simulink library "see_saw_princess"  (R2013b)
settings: Solver=ode45  StartTime=0.0  StopTime=10.0  RelTol=1e-3
undefined symbols (not defined in the file): DiscIntNeverNeededParam, K, R
libraries: legonxtlib x4
settings Model: Creator=mbiesiad  LastModifiedBy=pvinnako

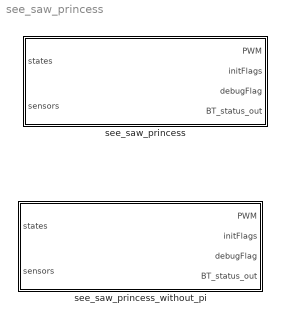
== system see_saw_princess ==
  see_saw_princess : Stateflow chart  TreatAsAtomicUnit=on
  see_saw_princess_without_pi : Stateflow chart  TreatAsAtomicUnit=on

== system see_saw_princess/see_saw_princess/see_saw_mode.DispVar ==
  Var : Inport  OutDataTypeStr=single  PortDimensions=1
  f : TriggerPort  TriggerType=function-call
      settings: CopyFcn=Stateflow.SLINSF.SimulinkMan.removeBlockPreDeleteFcn  PreDeleteFcn=Stateflow.SLINSF.SimulinkMan.unsafePredeleteFcn
  Gain : Gain  Gain=100
  LCD : legonxtlib/LCD  slcdStr=Light  slcdLine=2  slcdFormat=Decimal
  wires:
  Gain/1 -> LCD/1
  Var/1 -> Gain/1

== system see_saw_princess/see_saw_princess/see_saw_mode.Speak ==
  f : TriggerPort  TriggerType=function-call
      settings: CopyFcn=Stateflow.SLINSF.SimulinkMan.removeBlockPreDeleteFcn  PreDeleteFcn=Stateflow.SLINSF.SimulinkMan.unsafePredeleteFcn
  Constant : Constant  Value=50
  Speaker : legonxtlib/Speaker  sinputMode=Volume only  sspeakerFreq=800  sspeakerVolume=50  sspeakerDuration=100
  wires:
  Constant/1 -> Speaker/1

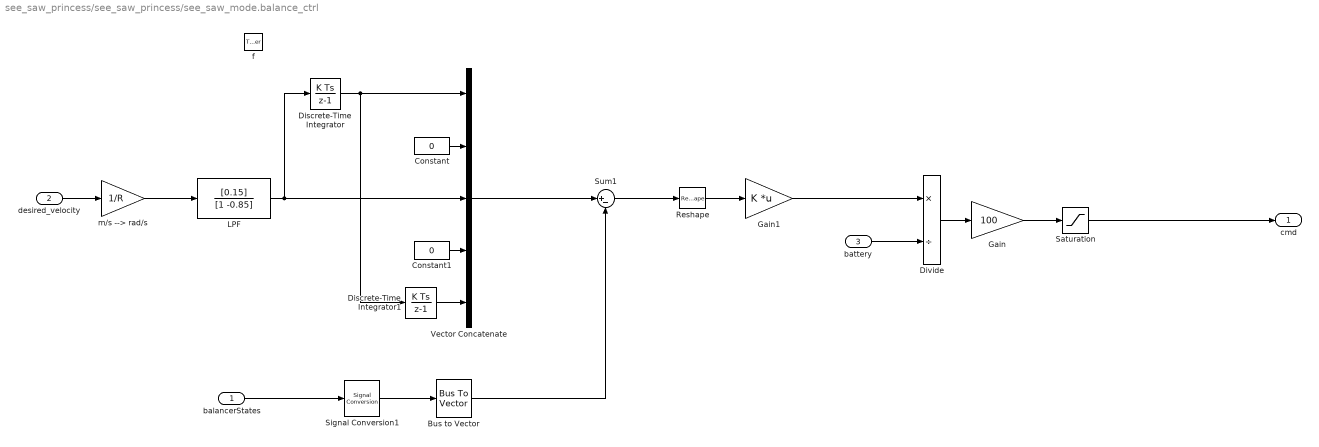
== system see_saw_princess/see_saw_princess/see_saw_mode.balance_ctrl ==
  balancerStates : Inport  OutDataTypeStr=Bus: Balancer_States_Bus  PortDimensions=1
  desired_velocity : Inport  Port=2  OutDataTypeStr=single  PortDimensions=1  BusOutputAsStruct=on
  battery : Inport  Port=3  OutDataTypeStr=double  PortDimensions=1
  f : TriggerPort  TriggerType=function-call
      settings: CopyFcn=Stateflow.SLINSF.SimulinkMan.removeBlockPreDeleteFcn  PreDeleteFcn=Stateflow.SLINSF.SimulinkMan.unsafePredeleteFcn
  Bus to Vector : BusToVector
  Constant : Constant  Value=0  OutDataTypeStr=single
  Constant1 : Constant  Value=0  OutDataTypeStr=single
  Discrete-Time Integrator : DiscreteIntegrator  SampleTime=-1  ICPrevOutput=DiscIntNeverNeededParam  ICPrevScaledInput=DiscIntNeverNeededParam
  Discrete-Time Integrator1 : DiscreteIntegrator  SampleTime=-1  ICPrevOutput=DiscIntNeverNeededParam  ICPrevScaledInput=DiscIntNeverNeededParam
  Divide : Product  Inputs=*/
  Gain : Gain  Gain=100
  Gain1 : Gain  Gain=K  Multiplication=Matrix(K*u)
  LPF : DiscreteFilter  Numerator=[0.15]  Denominator=[1 -0.85]
  Reshape : Reshape  OutputDimensionality=Column vector (2-D)
  Saturation : Saturate  UpperLimit=100  LowerLimit=-100  OutDataTypeStr=single
  Signal Conversion1 : SignalConversion  ConversionOutput=Virtual bus
  Sum1 : Sum  Inputs=|+-
  Vector Concatenate : Concatenate  NumInputs=5
  m/s --> rad/s : Gain  Gain=1/R
  cmd : Outport  OutDataTypeStr=single  PortDimensions=1  InitialOutput=0
  wires:
  Discrete-Time Integrator1/1 -> Vector Concatenate/5
  Discrete-Time Integrator/1 -> Vector Concatenate/1, Discrete-Time Integrator1/1
  Constant1/1 -> Vector Concatenate/4
  LPF/1 -> Vector Concatenate/3, Discrete-Time Integrator/1
  Constant/1 -> Vector Concatenate/2
  m/s --> rad/s/1 -> LPF/1
  Signal Conversion1/1 -> Bus to Vector/1
  Divide/1 -> Gain/1
  Gain/1 -> Saturation/1
  Gain1/1 -> Divide/1
  Saturation/1 -> cmd/1
  battery/1 -> Divide/2
  Vector Concatenate/1 -> Sum1/1
  balancerStates/1 -> Signal Conversion1/1
  Bus to Vector/1 -> Sum1/2
  desired_velocity/1 -> m/s --> rad/s/1
  Sum1/1 -> Reshape/1
  Reshape/1 -> Gain1/1

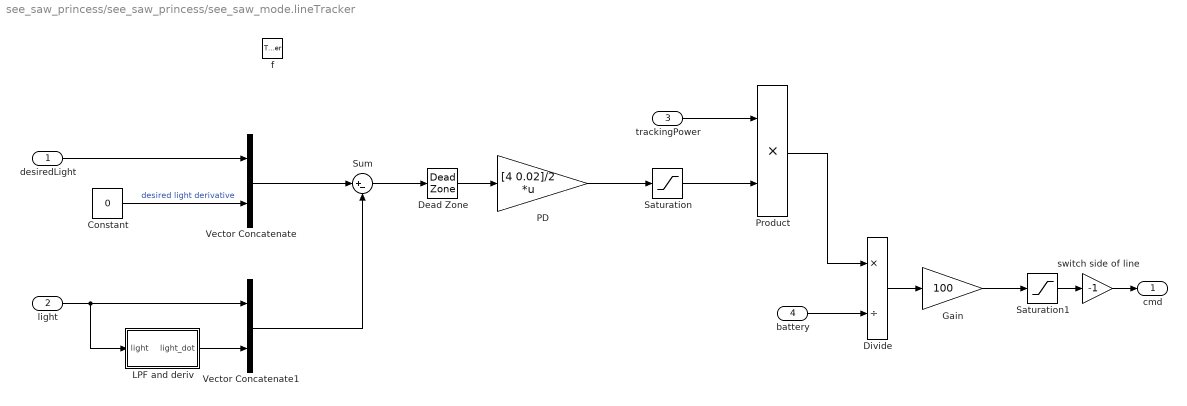
== system see_saw_princess/see_saw_princess/see_saw_mode.lineTracker ==
  desiredLight : Inport  OutDataTypeStr=single  PortDimensions=1
  light : Inport  Port=2  OutDataTypeStr=single  PortDimensions=1
  trackingPower : Inport  Port=3  OutDataTypeStr=single  PortDimensions=1
  battery : Inport  Port=4  OutDataTypeStr=double  PortDimensions=1
  f : TriggerPort  TriggerType=function-call
      settings: CopyFcn=Stateflow.SLINSF.SimulinkMan.removeBlockPreDeleteFcn  PreDeleteFcn=Stateflow.SLINSF.SimulinkMan.unsafePredeleteFcn
  Constant : Constant  Value=0  OutDataTypeStr=single
  Dead Zone : DeadZone  LowerValue=-0.02  UpperValue=0.02  SaturateOnIntegerOverflow=on
  Divide : Product  Inputs=*/
  Gain : Gain  Gain=100
  LPF and deriv : Subsystem
  PD : Gain  Gain="[4  0.02]/2"  Multiplication=Matrix(K*u)
  Product : Product
  Saturation : Saturate  UpperLimit=6  LowerLimit=-6
  Saturation1 : Saturate  UpperLimit=100  LowerLimit=-100  OutDataTypeStr=single
  Sum : Sum  Inputs=|+-
  Vector Concatenate : Concatenate
  Vector Concatenate1 : Concatenate
  switch side of line : Gain  Gain=-1
  cmd : Outport  OutDataTypeStr=single  PortDimensions=1
  wires:
  Saturation1/1 -> switch side of line/1
  Divide/1 -> Gain/1
  Gain/1 -> Saturation1/1
  battery/1 -> Divide/2
  Product/1 -> Divide/1
  trackingPower/1 -> Product/1
  Saturation/1 -> Product/2
  PD/1 -> Saturation/1
  Dead Zone/1 -> PD/1
  Sum/1 -> Dead Zone/1
  Vector Concatenate1/1 -> Sum/2
  Vector Concatenate/1 -> Sum/1
  light/1 -> Vector Concatenate1/1, LPF and deriv/1(light)
  LPF and deriv/1(light_dot) -> Vector Concatenate1/2
  Constant/1 -> Vector Concatenate/2  "desired light derivative"
  desiredLight/1 -> Vector Concatenate/1
  switch side of line/1 -> cmd/1

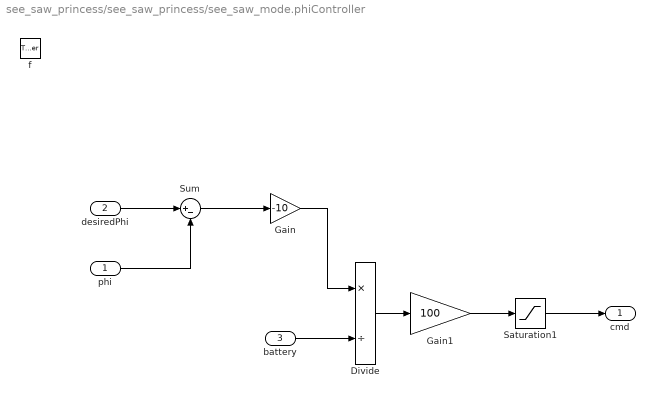
== system see_saw_princess/see_saw_princess/see_saw_mode.phiController ==
  phi : Inport  OutDataTypeStr=single  PortDimensions=1
  desiredPhi : Inport  Port=2  OutDataTypeStr=single  PortDimensions=1
  battery : Inport  Port=3  OutDataTypeStr=double  PortDimensions=1
  f : TriggerPort  TriggerType=function-call
      settings: CopyFcn=Stateflow.SLINSF.SimulinkMan.removeBlockPreDeleteFcn  PreDeleteFcn=Stateflow.SLINSF.SimulinkMan.unsafePredeleteFcn
  Divide : Product  Inputs=*/
  Gain : Gain  Gain=-10
  Gain1 : Gain  Gain=100
  Saturation1 : Saturate  UpperLimit=100  LowerLimit=-100  OutDataTypeStr=single
  Sum : Sum  Inputs=|+-
  cmd : Outport
  wires:
  Saturation1/1 -> cmd/1
  Gain/1 -> Divide/1
  Divide/1 -> Gain1/1
  Gain1/1 -> Saturation1/1
  battery/1 -> Divide/2
  Sum/1 -> Gain/1
  phi/1 -> Sum/2
  desiredPhi/1 -> Sum/1

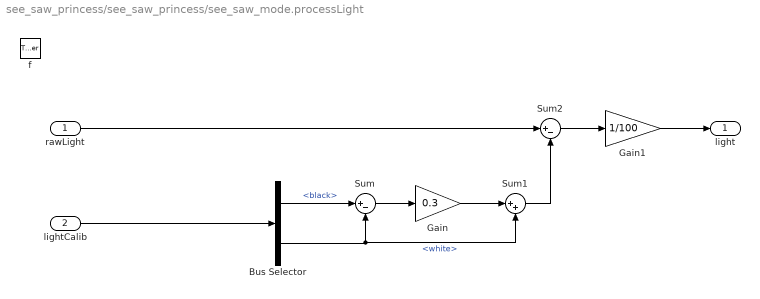
== system see_saw_princess/see_saw_princess/see_saw_mode.processLight ==
  rawLight : Inport  OutDataTypeStr=single  PortDimensions=1
  lightCalib : Inport  Port=2  OutDataTypeStr=Bus: Light_Bus  PortDimensions=1
  f : TriggerPort  TriggerType=function-call
      settings: CopyFcn=Stateflow.SLINSF.SimulinkMan.removeBlockPreDeleteFcn  PreDeleteFcn=Stateflow.SLINSF.SimulinkMan.unsafePredeleteFcn
  Bus Selector : BusSelector  OutputSignals=black,white
  Gain : Gain  Gain=0.3
  Gain1 : Gain  Gain=1/100
  Sum : Sum  Inputs=|+-
  Sum1 : Sum  Inputs=|++
  Sum2 : Sum  Inputs=|+-
  light : Outport
  wires:
  Gain1/1 -> light/1
  Sum2/1 -> Gain1/1
  Sum1/1 -> Sum2/2
  rawLight/1 -> Sum2/1
  Gain/1 -> Sum1/1
  Sum/1 -> Gain/1
  Bus Selector/2 -> Sum/2, Sum1/2  "<white>"
  Bus Selector/1 -> Sum/1  "<black>"
  lightCalib/1 -> Bus Selector/1

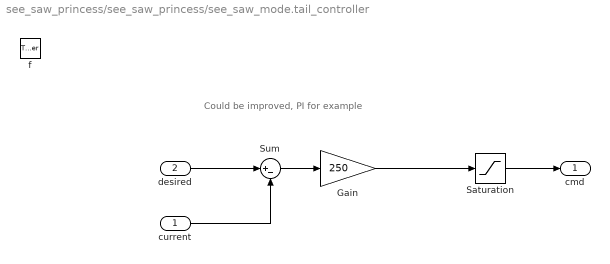
== system see_saw_princess/see_saw_princess/see_saw_mode.tail_controller ==
  note: Could be improved, PI for example
  current : Inport  OutDataTypeStr=single  PortDimensions=1
  desired : Inport  Port=2  OutDataTypeStr=single  PortDimensions=1
  f : TriggerPort  TriggerType=function-call
      settings: CopyFcn=Stateflow.SLINSF.SimulinkMan.removeBlockPreDeleteFcn  PreDeleteFcn=Stateflow.SLINSF.SimulinkMan.unsafePredeleteFcn
  Gain : Gain  Gain=250
  Saturation : Saturate  UpperLimit=100  LowerLimit=-100  OutDataTypeStr=single
  Sum : Sum  Inputs=|+-
  cmd : Outport  OutDataTypeStr=single  PortDimensions=1  InitialOutput=0
  wires:
  Saturation/1 -> cmd/1
  Gain/1 -> Saturation/1
  desired/1 -> Sum/1
  current/1 -> Sum/2
  Sum/1 -> Gain/1

== system see_saw_princess/see_saw_princess_without_pi/see_saw_mode.DispVar ==
  Var : Inport  OutDataTypeStr=single  PortDimensions=1
  f : TriggerPort  TriggerType=function-call
      settings: CopyFcn=Stateflow.SLINSF.SimulinkMan.removeBlockPreDeleteFcn  PreDeleteFcn=Stateflow.SLINSF.SimulinkMan.unsafePredeleteFcn
  Gain : Gain  Gain=100
  LCD : legonxtlib/LCD  slcdStr=Light  slcdLine=2  slcdFormat=Decimal
  wires:
  Var/1 -> Gain/1
  Gain/1 -> LCD/1

== system see_saw_princess/see_saw_princess_without_pi/see_saw_mode.Speak ==
  f : TriggerPort  TriggerType=function-call
      settings: CopyFcn=Stateflow.SLINSF.SimulinkMan.removeBlockPreDeleteFcn  PreDeleteFcn=Stateflow.SLINSF.SimulinkMan.unsafePredeleteFcn
  Constant : Constant  Value=50
  Speaker : legonxtlib/Speaker  sinputMode=Volume only  sspeakerFreq=800  sspeakerVolume=50  sspeakerDuration=100
  wires:
  Constant/1 -> Speaker/1

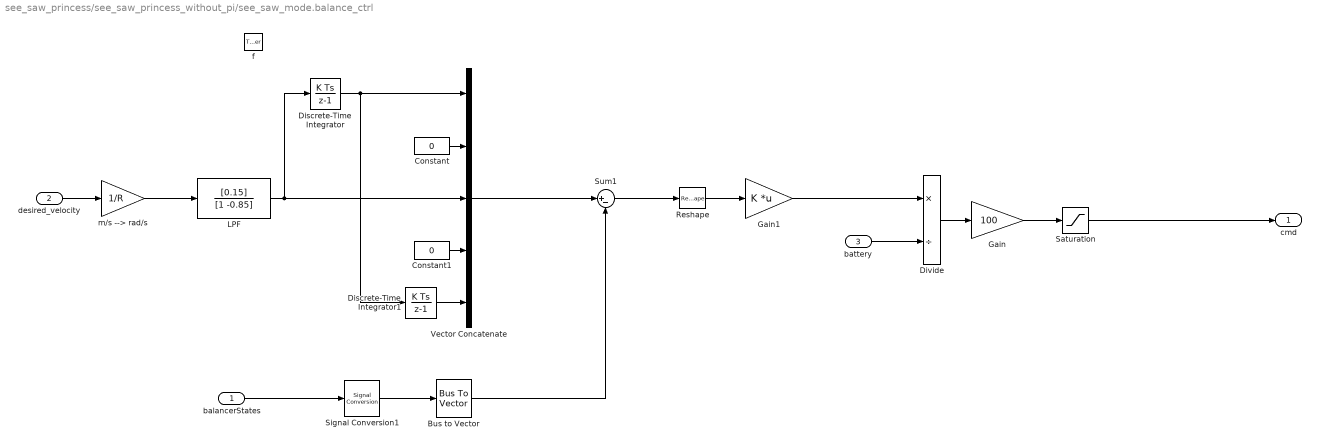
== system see_saw_princess/see_saw_princess_without_pi/see_saw_mode.balance_ctrl ==
  balancerStates : Inport  OutDataTypeStr=Bus: Balancer_States_Bus  PortDimensions=1
  desired_velocity : Inport  Port=2  OutDataTypeStr=single  PortDimensions=1  BusOutputAsStruct=on
  battery : Inport  Port=3  OutDataTypeStr=double  PortDimensions=1
  f : TriggerPort  TriggerType=function-call
      settings: CopyFcn=Stateflow.SLINSF.SimulinkMan.removeBlockPreDeleteFcn  PreDeleteFcn=Stateflow.SLINSF.SimulinkMan.unsafePredeleteFcn
  Bus to Vector : BusToVector
  Constant : Constant  Value=0  OutDataTypeStr=single
  Constant1 : Constant  Value=0  OutDataTypeStr=single
  Discrete-Time Integrator : DiscreteIntegrator  SampleTime=-1  ICPrevOutput=DiscIntNeverNeededParam  ICPrevScaledInput=DiscIntNeverNeededParam
  Discrete-Time Integrator1 : DiscreteIntegrator  SampleTime=-1  ICPrevOutput=DiscIntNeverNeededParam  ICPrevScaledInput=DiscIntNeverNeededParam
  Divide : Product  Inputs=*/
  Gain : Gain  Gain=100
  Gain1 : Gain  Gain=K  Multiplication=Matrix(K*u)
  LPF : DiscreteFilter  Numerator=[0.15]  Denominator=[1 -0.85]
  Reshape : Reshape  OutputDimensionality=Column vector (2-D)
  Saturation : Saturate  UpperLimit=100  LowerLimit=-100  OutDataTypeStr=single
  Signal Conversion1 : SignalConversion  ConversionOutput=Virtual bus
  Sum1 : Sum  Inputs=|+-
  Vector Concatenate : Concatenate  NumInputs=5
  m/s --> rad/s : Gain  Gain=1/R
  cmd : Outport  OutDataTypeStr=single  PortDimensions=1  InitialOutput=0
  wires:
  Reshape/1 -> Gain1/1
  Sum1/1 -> Reshape/1
  desired_velocity/1 -> m/s --> rad/s/1
  Bus to Vector/1 -> Sum1/2
  balancerStates/1 -> Signal Conversion1/1
  Vector Concatenate/1 -> Sum1/1
  battery/1 -> Divide/2
  Saturation/1 -> cmd/1
  Gain1/1 -> Divide/1
  Gain/1 -> Saturation/1
  Divide/1 -> Gain/1
  Signal Conversion1/1 -> Bus to Vector/1
  m/s --> rad/s/1 -> LPF/1
  Constant/1 -> Vector Concatenate/2
  LPF/1 -> Discrete-Time Integrator/1, Vector Concatenate/3
  Constant1/1 -> Vector Concatenate/4
  Discrete-Time Integrator/1 -> Discrete-Time Integrator1/1, Vector Concatenate/1
  Discrete-Time Integrator1/1 -> Vector Concatenate/5

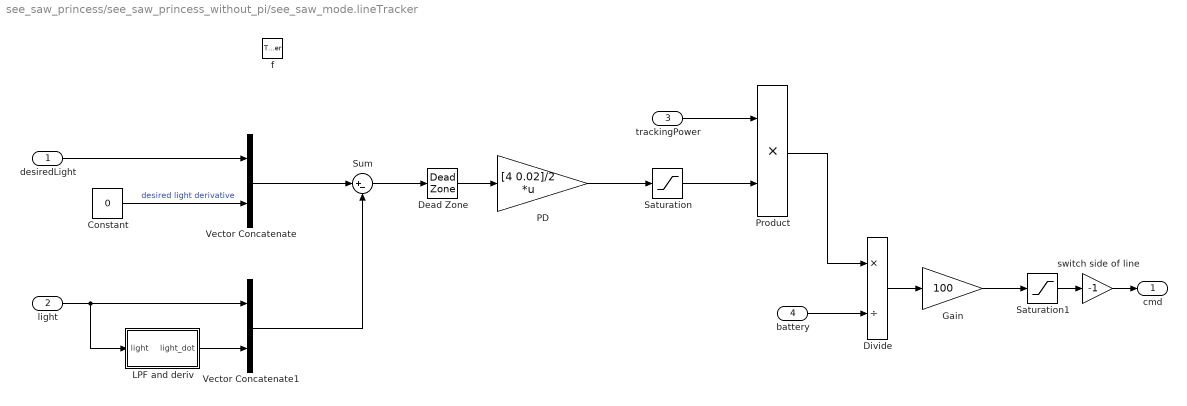
== system see_saw_princess/see_saw_princess_without_pi/see_saw_mode.lineTracker ==
  desiredLight : Inport  OutDataTypeStr=single  PortDimensions=1
  light : Inport  Port=2  OutDataTypeStr=single  PortDimensions=1
  trackingPower : Inport  Port=3  OutDataTypeStr=single  PortDimensions=1
  battery : Inport  Port=4  OutDataTypeStr=double  PortDimensions=1
  f : TriggerPort  TriggerType=function-call
      settings: CopyFcn=Stateflow.SLINSF.SimulinkMan.removeBlockPreDeleteFcn  PreDeleteFcn=Stateflow.SLINSF.SimulinkMan.unsafePredeleteFcn
  Constant : Constant  Value=0  OutDataTypeStr=single
  Dead Zone : DeadZone  LowerValue=-0.02  UpperValue=0.02  SaturateOnIntegerOverflow=on
  Divide : Product  Inputs=*/
  Gain : Gain  Gain=100
  LPF and deriv : Subsystem
  PD : Gain  Gain="[4  0.02]/2"  Multiplication=Matrix(K*u)
  Product : Product
  Saturation : Saturate  UpperLimit=6  LowerLimit=-6
  Saturation1 : Saturate  UpperLimit=100  LowerLimit=-100  OutDataTypeStr=single
  Sum : Sum  Inputs=|+-
  Vector Concatenate : Concatenate
  Vector Concatenate1 : Concatenate
  switch side of line : Gain  Gain=-1
  cmd : Outport  OutDataTypeStr=single  PortDimensions=1
  wires:
  switch side of line/1 -> cmd/1
  desiredLight/1 -> Vector Concatenate/1
  Constant/1 -> Vector Concatenate/2  "desired light derivative"
  LPF and deriv/1(light_dot) -> Vector Concatenate1/2
  light/1 -> LPF and deriv/1(light), Vector Concatenate1/1
  Vector Concatenate/1 -> Sum/1
  Vector Concatenate1/1 -> Sum/2
  Sum/1 -> Dead Zone/1
  Dead Zone/1 -> PD/1
  PD/1 -> Saturation/1
  Saturation/1 -> Product/2
  trackingPower/1 -> Product/1
  Product/1 -> Divide/1
  battery/1 -> Divide/2
  Gain/1 -> Saturation1/1
  Divide/1 -> Gain/1
  Saturation1/1 -> switch side of line/1

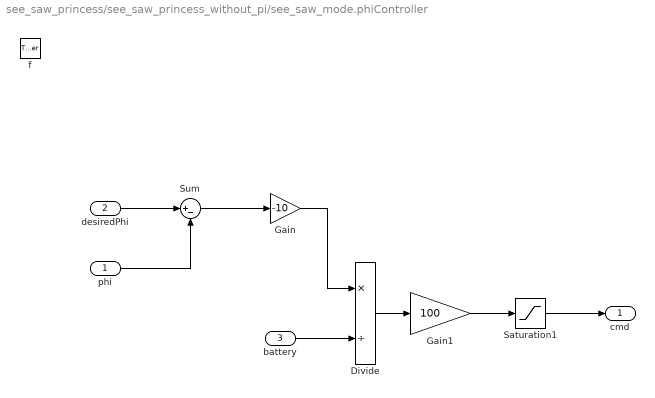
== system see_saw_princess/see_saw_princess_without_pi/see_saw_mode.phiController ==
  phi : Inport  OutDataTypeStr=single  PortDimensions=1
  desiredPhi : Inport  Port=2  OutDataTypeStr=single  PortDimensions=1
  battery : Inport  Port=3  OutDataTypeStr=double  PortDimensions=1
  f : TriggerPort  TriggerType=function-call
      settings: CopyFcn=Stateflow.SLINSF.SimulinkMan.removeBlockPreDeleteFcn  PreDeleteFcn=Stateflow.SLINSF.SimulinkMan.unsafePredeleteFcn
  Divide : Product  Inputs=*/
  Gain : Gain  Gain=-10
  Gain1 : Gain  Gain=100
  Saturation1 : Saturate  UpperLimit=100  LowerLimit=-100  OutDataTypeStr=single
  Sum : Sum  Inputs=|+-
  cmd : Outport
  wires:
  desiredPhi/1 -> Sum/1
  phi/1 -> Sum/2
  Sum/1 -> Gain/1
  battery/1 -> Divide/2
  Gain1/1 -> Saturation1/1
  Divide/1 -> Gain1/1
  Gain/1 -> Divide/1
  Saturation1/1 -> cmd/1

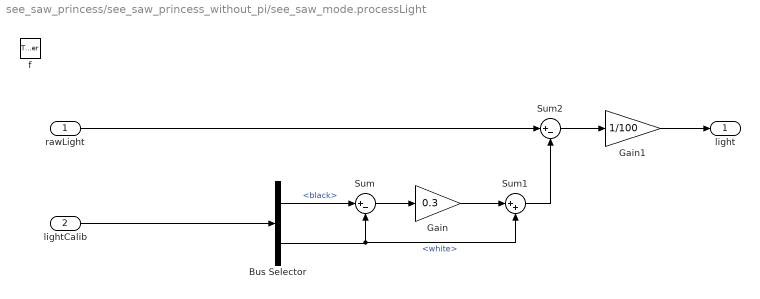
== system see_saw_princess/see_saw_princess_without_pi/see_saw_mode.processLight ==
  rawLight : Inport  OutDataTypeStr=single  PortDimensions=1
  lightCalib : Inport  Port=2  OutDataTypeStr=Bus: Light_Bus  PortDimensions=1
  f : TriggerPort  TriggerType=function-call
      settings: CopyFcn=Stateflow.SLINSF.SimulinkMan.removeBlockPreDeleteFcn  PreDeleteFcn=Stateflow.SLINSF.SimulinkMan.unsafePredeleteFcn
  Bus Selector : BusSelector  OutputSignals=black,white
  Gain : Gain  Gain=0.3
  Gain1 : Gain  Gain=1/100
  Sum : Sum  Inputs=|+-
  Sum1 : Sum  Inputs=|++
  Sum2 : Sum  Inputs=|+-
  light : Outport
  wires:
  lightCalib/1 -> Bus Selector/1
  Bus Selector/1 -> Sum/1  "<black>"
  Bus Selector/2 -> Sum1/2, Sum/2  "<white>"
  Sum/1 -> Gain/1
  Gain/1 -> Sum1/1
  rawLight/1 -> Sum2/1
  Sum1/1 -> Sum2/2
  Sum2/1 -> Gain1/1
  Gain1/1 -> light/1

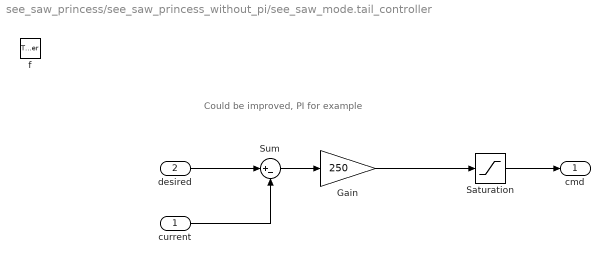
== system see_saw_princess/see_saw_princess_without_pi/see_saw_mode.tail_controller ==
  note: Could be improved, PI for example
  current : Inport  OutDataTypeStr=single  PortDimensions=1
  desired : Inport  Port=2  OutDataTypeStr=single  PortDimensions=1
  f : TriggerPort  TriggerType=function-call
      settings: CopyFcn=Stateflow.SLINSF.SimulinkMan.removeBlockPreDeleteFcn  PreDeleteFcn=Stateflow.SLINSF.SimulinkMan.unsafePredeleteFcn
  Gain : Gain  Gain=250
  Saturation : Saturate  UpperLimit=100  LowerLimit=-100  OutDataTypeStr=single
  Sum : Sum  Inputs=|+-
  cmd : Outport  OutDataTypeStr=single  PortDimensions=1  InitialOutput=0
  wires:
  Sum/1 -> Gain/1
  current/1 -> Sum/2
  desired/1 -> Sum/1
  Gain/1 -> Saturation/1
  Saturation/1 -> cmd/1

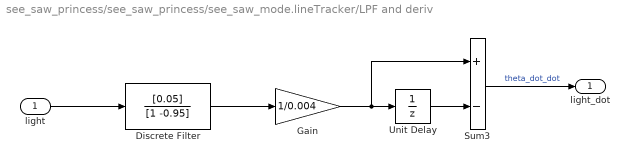
== system see_saw_princess/see_saw_princess/see_saw_mode.lineTracker/LPF and deriv ==
  light : Inport
  Discrete Filter : DiscreteFilter  Numerator=[0.05]  Denominator=[1 -0.95]
  Gain : Gain  Gain=1/0.004
  Sum3 : Sum  Inputs=+-
  Unit Delay : UnitDelay  SampleTime=-1
  light_dot : Outport
  wires:
  Unit Delay/1 -> Sum3/2
  Gain/1 -> Unit Delay/1, Sum3/1
  Sum3/1 -> light_dot/1  "theta_dot_dot"
  Discrete Filter/1 -> Gain/1
  light/1 -> Discrete Filter/1

== system see_saw_princess/see_saw_princess_without_pi/see_saw_mode.lineTracker/LPF and deriv ==
  light : Inport
  Discrete Filter : DiscreteFilter  Numerator=[0.05]  Denominator=[1 -0.95]
  Gain : Gain  Gain=1/0.004
  Sum3 : Sum  Inputs=+-
  Unit Delay : UnitDelay  SampleTime=-1
  light_dot : Outport
  wires:
  light/1 -> Discrete Filter/1
  Discrete Filter/1 -> Gain/1
  Sum3/1 -> light_dot/1  "theta_dot_dot"
  Gain/1 -> Sum3/1, Unit Delay/1
  Unit Delay/1 -> Sum3/2

== stateflow chart see_saw_princess/see_saw_princess ==
  state see_saw_mode
    entry:
    desired_tail = single(1.6);
    during:
    normalizedLight = processLight(sensors.light,lightCalib);
    PWM.tail = tail_controller(sensors.theta_T, desired_tail);
    DispVar(normalizedLight);
    state Pause
      entry:
      debugFlag = uint16(601);
    state light = processLight(rawLight,lightCalib) [function]
    state StandUp
      entry: debugFlag = uint16(602);
      initFlags.theta = single(1);
      initFlags.gyroReset = single(1);
      during:
      desired_tail = desired_tail + single(0.0008);
    state cmd = phiController(phi,desiredPhi,battery) [function]
    state Balancing
      state SeesawLogic [parallel]
        settings: executionOrder=1
        state StationnaryBalance
          entry:
          debugFlag = uint16(603);
          desired_tail = single(0.5);
          initFlags.theta = single(0);
          initFlags.gyroReset = single(0);
          desired_states = balancerStates_Bus0;
          phi0 = states.phi;
          desired_phi = phi0;
          during:
          turningPWM = phiController(states.phi,desired_phi,sensors.battery);
          exit:
          turningPWM = single(0);
        state Approach
          entry:
          debugFlag = uint16(604);
          during:
          turningPWM = lineTracker(single(-0.3), normalizedLight, single(1.3), sensors.battery);
          exit:
          turningPWM = single(0);
          state StartWalking
            entry:
            debugFlag = uint16(605);
            des_vel = single(0.02);
            during:
            des_vel = des_vel+single(0.00024);
          state Detect
            state Walk
              entry: debugFlag = uint16(6051);
              during:
              des_vel = des_vel+single(0.00024);
            state Walk1
              entry: debugFlag = uint16(6052);
            Walk -> Walk1 : [des_vel >= single(0.1)]
          (default) -> StartWalking
          StartWalking -> Walk : [states.balancerStates.theta>single(3)]
        state Seesaw
          entry:
          phi0 = states.phi;
          desired_phi = phi0;
          Speak;
          exit:
          turningPWM = single(0);
          BT_status_out = single(42);
          note: % For now I store theta_ref when we receive the bluetooth signal.
              | Eventually one state needs to be added to sear for the ramp
              | and we should store the ref when the ramp is detected.
          state JumpOnIt
            entry:
            debugFlag = uint16(606);
            theta_ref = states.balancerStates.theta;
            des_vel = single(0.16);
            du:
            turningPWM = phiController(states.phi,desired_phi, sensors.battery);
          state ForPhi
            state GoingUP
              en:
              debugFlag = uint16(607);
              des_vel = single(0.1);
              du:
              turningPWM = phiController(states.phi,desired_phi, sensors.battery)+...
              single(3)*lineTracker(single(0.15), normalizedLight, single(1), sensors.battery);
              ex:
              des_vel = single(0);
            state WaitForMario
              en:
              debugFlag = uint16(608);
              des_vel = single(0);
              BT_status_out = single(40);
              du:
              turningPWM =phiController(states.phi,desired_phi, sensors.battery)
            state MoveForward
              en:
              debugFlag = uint16(609);
              des_vel = single(0.005);
              du:
              turningPWM = phiController(states.phi,desired_phi, sensors.battery)+...
              single(3)*lineTracker(single(0.3), normalizedLight, single(1), sensors.battery);
              ex:
              %des_vel = single(0.01);
              state Vel1
                du: des_vel = des_vel + single(0.00024);
              state Vel
                entry:
                des_vel = single(0.06)
                BT_status_out = single(41);
              (default) -> see_saw_mode.Balancing.SeesawLogic.Seesaw.ForPhi.MoveForward.Vel1
              see_saw_mode.Balancing.SeesawLogic.Seesaw.ForPhi.MoveForward.Vel1 -> see_saw_mode.Balancing.SeesawLogic.Seesaw.ForPhi.MoveForward.Vel : [des_vel >= single(0.06)]
            GoingUP -> WaitForMario : [states.balancerStates.theta >= theta_ref + single(5)]
            WaitForMario -> MoveForward : [sensors.BT_status_in == single(52)]
                | {Speak;}
          state Wait
            entry:
            debugFlag = uint16(611);
            des_vel = single(0);
            during:
            turningPWM = phiController(states.phi,desired_phi, sensors.battery);
            exit: des_vel = single(0.05);
          state Stop
            entry:
            debugFlag = uint16(612);
            BT_status_out = single(104);
            du:
            turningPWM = single(1.1)*lineTracker(single(0.3), normalizedLight, single(1), sensors.battery)+single(1)*phiController(states.phi,desired_phi,sensors.battery);
            %turningPWM = phiController(states.phi,desired_phi, sensors.battery);
          state FindingLine
            en:
            turningPWM = phiController(states.phi,desired_phi,sensors.battery);
            des_vel = single(0);
            state TurnAndBackup
              entry:
              debugFlag = uint16(612);
              BT_status_out = single(4);
              du:
              desired_phi = desired_phi + single(0.003);
              des_vel = single(0);
              turningPWM = phiController(states.phi,desired_phi,sensors.battery);
            state HuntLine
              entry: debugFlag = uint16(613)
              desired_phi = states.phi;
              theta_ref_2 = states.balancerStates.theta;
              du: turningPWM = phiController(states.phi,desired_phi,sensors.battery);
              state GoForward
                en:  des_vel= single(0.04);
                entry: debugFlag = uint16(6131);
              state BackUpB
                en: des_vel = single(-0.04)
                entry: debugFlag = uint16(6132);
              BackUpB -> GoForward : [states.balancerStates.theta <= theta_ref_2 - single(3) ]
              (default) -> BackUpB
              GoForward -> BackUpB : [states.balancerStates.theta >= theta_ref_2 + single(3) ]
            state TurnAndBackup1
              entry:
              Speak
              debugFlag = uint16(614);
              BT_status_out = single(4);
              des_vel = des_vel / single(3);
              du:
              desired_phi = desired_phi - single(0.003);
              turningPWM = phiController(states.phi,desired_phi,sensors.battery);
            state GoForwardUntilLine
              en:
              Speak;
              debugFlag = uint16(615)
              des_vel = single(0);
            (default) -> TurnAndBackup
            TurnAndBackup -> HuntLine : [phi0+states.phi > single(1.6)]
            HuntLine -> TurnAndBackup1 : [normalizedLight >= single(0.5)]
            TurnAndBackup1 -> GoForwardUntilLine : [phi0+states.phi < single(0.7)]
            GoForwardUntilLine -> ? : after(1,sec)
          state RaceDone
            entry: debugFlag = uint16(613);
            du: turningPWM = phiController(states.phi,desired_phi, sensors.battery)+...
            single(3)*lineTracker(single(-0.3), normalizedLight, single(1), sensors.battery);
            state Vel
            state Vel1
              du: des_vel = des_vel + single(0.00024);
            see_saw_mode.Balancing.SeesawLogic.Seesaw.RaceDone.Vel1 -> see_saw_mode.Balancing.SeesawLogic.Seesaw.RaceDone.Vel : [des_vel >= single(0.15)]
            (default) -> see_saw_mode.Balancing.SeesawLogic.Seesaw.RaceDone.Vel1
          state FoundLine
            entry: debugFlag = uint16(614);
            du: turningPWM = lineTracker(single(-0.3), normalizedLight, single(1.3), sensors.battery);
            state Vel3
            state Vel2
              du: des_vel = des_vel + single(0.00024);
            Vel2 -> Vel3 : [des_vel >= single(0.15)]
            (default) -> Vel2
          (default) -> JumpOnIt
          JumpOnIt -> GoingUP : [states.balancerStates.theta >= theta_ref+single(1.6)]
          MoveForward -> Wait : [sensors.BT_status_in == single(53)]
              | {Speak;}
          Wait -> see_saw_mode.Balancing.SeesawLogic.Seesaw.Stop : [sensors.BT_status_in == single(54)]
              | {Speak;}
          see_saw_mode.Balancing.SeesawLogic.Seesaw.Stop -> RaceDone : [states.balancerStates.theta >= theta_ref + single(30)]
          RaceDone -> FoundLine [order 2] : [normalizedLight > single(0.4)]
        (default) -> StationnaryBalance
        StationnaryBalance -> Approach : [sensors.BT_status_in == single(51)]
            | {Speak;}
        Detect -> Seesaw : [states.balancerStates.theta_dot<single(0)]
      state After [parallel]
        during:
        forwardPWM = balance_ctrl(states.balancerStates, des_vel ,sensors.battery)
        PWM.left = forwardPWM + turningPWM;
        PWM.right = forwardPWM - turningPWM;
        settings: executionOrder=2
    state cmd = lineTracker(desiredLight,light,trackingPower,battery) [function]
    state Speak [function]
    state cmd = tail_controller(current,desired) [function]
    state cmd = balance_ctrl(balancerStates,desired_velocity,battery) [function]
    state DispVar(Var) [function]
    state SitDown
      state Stop
        during:
        during:
        forwardPWM = balance_ctrl(states.balancerStates, des_vel ,sensors.battery)
        PWM.left = forwardPWM;
        PWM.right = forwardPWM;
        desired_tail = single(1.6); %radian
      state Kick
        entry:
        PWM.left = single(100)
        PWM.right = single(100);
        exit:
        PWM.left = single(0)
        PWM.right = single(0);
      state Done
        entry:
        debugFlag = uint16(402);
        PWM.left = single(0); PWM.right = single(0);
        %current_mode_status = OperationModeStatusEnum.SUCCESSFULLY_COMPLETED;
      (default) -> see_saw_mode.SitDown.Stop
      see_saw_mode.SitDown.Stop -> Kick : after(0.5,sec)
      Kick -> Done : after(0.2,sec)
    (default) -> Pause
    Pause -> StandUp : [sensors.BT_status_in == single(50)]
        | {Speak;}
    StandUp -> Balancing : [desired_tail >=single(2.0) && sensors.theta_T >= single(2.0)]
    RaceDone -> SitDown [order 1] : [states.balancerStates.theta >= theta_ref + single(70)]
    FoundLine -> SitDown : [states.balancerStates.theta >= theta_ref + single(70)]
  data: rawLight function_input single size=1; lightCalib function_input Bus: Light_Bus size=1; light function_output; cmd function_output; phi function_input single size=1; desiredPhi function_input single size=1; battery function_input double size=1; cmd function_output single size=1; desiredLight function_input single size=1; light function_input single size=1; trackingPower function_input single size=1; battery function_input double size=1; current function_input single size=1; desired function_input single size=1; cmd function_output single size=1; balancerStates function_input Bus: Balancer_States_Bus size=1; desired_velocity function_input single size=1; battery function_input double size=1; cmd function_output single size=1; Var function_input single size=1; states input Bus: States_Bus size=1; sensors input Bus: Sensors_Bus size=1; PWM output Bus: PWM_bus size=1; initFlags output Bus: Init_Bus size=1; debugFlag output uint16 size=1; desired_states local Bus: Balancer_States_Bus size=1; desired_tail local single size=1; current_mode_status data_store_memory; balancerStates_Bus0 parameter Bus: Balancer_States_Bus size=1; lightCalib data_store_memory; normalizedLight local single size=1; des_vel local single size=1; theta_ref local single size=1; forwardPWM local single size=1; turningPWM local single size=1; BT_status_out output single size=1; phi0 local single size=1; desired_phi local single size=1; theta_ref_2 local

== stateflow chart see_saw_princess/see_saw_princess_without_pi ==
  state see_saw_mode
    entry:
    desired_tail = single(1.6);
    during:
    normalizedLight = processLight(sensors.light,lightCalib);
    PWM.tail = tail_controller(sensors.theta_T, desired_tail);
    DispVar(normalizedLight);
    state Pause
      entry:
      debugFlag = uint16(601);
    state light = processLight(rawLight,lightCalib) [function]
    state StandUp
      entry: debugFlag = uint16(602);
      initFlags.theta = single(1);
      initFlags.gyroReset = single(1);
      during:
      desired_tail = desired_tail + single(0.0008);
    state cmd = phiController(phi,desiredPhi,battery) [function]
    state Balancing
      state SeesawLogic [parallel]
        settings: executionOrder=1
        state StationnaryBalance
          entry:
          debugFlag = uint16(603);
          desired_tail = single(0.5);
          initFlags.theta = single(0);
          initFlags.gyroReset = single(0);
          desired_states = balancerStates_Bus0;
          phi0 = states.phi;
          desired_phi = phi0;
          during:
          turningPWM = phiController(states.phi,desired_phi,sensors.battery);
          exit:
          turningPWM = single(0);
        state Approach
          entry:
          debugFlag = uint16(604);
          during:
          turningPWM = lineTracker(single(-0.3), normalizedLight, single(1.3), sensors.battery);
          exit:
          turningPWM = single(0);
          state StartWalking
            entry:
            debugFlag = uint16(605);
            des_vel = single(0.02);
            during:
            des_vel = des_vel+single(0.00024);
          state Detect
            state Walk
              entry: debugFlag = uint16(6051);
              during:
              des_vel = des_vel+single(0.00024);
            state Walk1
              entry: debugFlag = uint16(6052);
            Walk -> Walk1 : [des_vel >= single(0.1)]
          (default) -> StartWalking
          StartWalking -> Walk : [states.balancerStates.theta>single(3)]
        state Seesaw
          entry:
          phi0 = states.phi;
          desired_phi = phi0;
          Speak;
          exit:
          turningPWM = single(0);
          note: % For now I store theta_ref when we receive the bluetooth signal.
              | Eventually one state needs to be added to sear for the ramp
              | and we should store the ref when the ramp is detected.
          state JumpOnIt
            entry:
            debugFlag = uint16(606);
            theta_ref = states.balancerStates.theta;
            des_vel = single(0.16);
            du:
            turningPWM = phiController(states.phi,desired_phi, sensors.battery);
          state ForPhi
            state GoingUP
              en:
              debugFlag = uint16(607);
              des_vel = single(0.1);
              du:
              turningPWM = phiController(states.phi,desired_phi, sensors.battery)+...
              single(3)*lineTracker(single(0.15), normalizedLight, single(1), sensors.battery);
              ex:
              des_vel = single(0);
            state WaitForMario
              en:
              debugFlag = uint16(608);
              des_vel = single(0);
              BT_status_out = single(102);
              du:
              turningPWM =phiController(states.phi,desired_phi, sensors.battery)
            state MoveForward
              en:
              debugFlag = uint16(609);
              des_vel = single(0.005);
              du:
              turningPWM = phiController(states.phi,desired_phi, sensors.battery)+...
              single(3)*lineTracker(single(0.3), normalizedLight, single(1), sensors.battery);
              ex:
              %des_vel = single(0.01);
              state Vel1
                du: des_vel = des_vel + single(0.00024);
              state Vel
                entry:
                des_vel = single(0.06)
                BT_status_out = single(103);
              (default) -> see_saw_mode.Balancing.SeesawLogic.Seesaw.ForPhi.MoveForward.Vel1
              see_saw_mode.Balancing.SeesawLogic.Seesaw.ForPhi.MoveForward.Vel1 -> see_saw_mode.Balancing.SeesawLogic.Seesaw.ForPhi.MoveForward.Vel : [des_vel >= single(0.06)]
            state WaitForMario2
              en:
              debugFlag = uint16(610);
              BT_status_out = single(103);
              du:
              turningPWM =phiController(states.phi,desired_phi, sensors.battery);
            GoingUP -> WaitForMario : [states.balancerStates.theta >= theta_ref + single(5)]
            WaitForMario -> MoveForward : [sensors.BT_status_in == single(3)]
          state Wait
            entry:
            debugFlag = uint16(611);
            des_vel = single(0);
            during:
            %turningPWM = single(1.1)*lineTracker(single(0.3), normalizedLight, single(1), sensors.battery)+single(1)*phiController(states.phi,desired_phi,sensors.battery);
            turningPWM = phiController(states.phi,desired_phi, sensors.battery);
            exit: des_vel = single(0.05);
          state Stop
            entry:
            debugFlag = uint16(612);
            BT_status_out = single(104);
            du:
            turningPWM = single(1.1)*lineTracker(single(0.3), normalizedLight, single(1), sensors.battery)+single(1)*phiController(states.phi,desired_phi,sensors.battery);
            %turningPWM = phiController(states.phi,desired_phi, sensors.battery);
          state FindingLine
            en:
            turningPWM = phiController(states.phi,desired_phi,sensors.battery);
            des_vel = single(0);
            state TurnAndBackup
              entry:
              debugFlag = uint16(612);
              BT_status_out = single(4);
              du:
              desired_phi = desired_phi + single(0.003);
              des_vel = single(0);
              turningPWM = phiController(states.phi,desired_phi,sensors.battery);
            state HuntLine
              entry: debugFlag = uint16(613)
              desired_phi = states.phi;
              theta_ref_2 = states.balancerStates.theta;
              du: turningPWM = phiController(states.phi,desired_phi,sensors.battery);
              state GoForward
                en:  des_vel= single(0.04);
                entry: debugFlag = uint16(6131);
              state BackUpB
                en: des_vel = single(-0.04)
                entry: debugFlag = uint16(6132);
              BackUpB -> GoForward : [states.balancerStates.theta <= theta_ref_2 - single(3) ]
              (default) -> BackUpB
              GoForward -> BackUpB : [states.balancerStates.theta >= theta_ref_2 + single(3) ]
            state TurnAndBackup1
              entry:
              Speak
              debugFlag = uint16(614);
              BT_status_out = single(4);
              des_vel = des_vel / single(3);
              du:
              desired_phi = desired_phi - single(0.003);
              turningPWM = phiController(states.phi,desired_phi,sensors.battery);
            state GoForwardUntilLine
              en:
              Speak;
              debugFlag = uint16(615)
              des_vel = single(0);
            (default) -> TurnAndBackup
            TurnAndBackup -> HuntLine : [phi0+states.phi > single(1.6)]
            HuntLine -> TurnAndBackup1 : [normalizedLight >= single(0.5)]
            TurnAndBackup1 -> GoForwardUntilLine : [phi0+states.phi < single(0.7)]
            GoForwardUntilLine -> ? : after(1,sec)
          state RaceDone
            entry: debugFlag = uint16(613);
            du: turningPWM = phiController(states.phi,desired_phi, sensors.battery)+...
            single(3)*lineTracker(single(-0.3), normalizedLight, single(1), sensors.battery);
            state Vel
            state Vel1
              du: des_vel = des_vel + single(0.00024);
            see_saw_mode.Balancing.SeesawLogic.Seesaw.RaceDone.Vel1 -> see_saw_mode.Balancing.SeesawLogic.Seesaw.RaceDone.Vel : [des_vel >= single(0.15)]
            (default) -> see_saw_mode.Balancing.SeesawLogic.Seesaw.RaceDone.Vel1
          state FoundLine
            entry: debugFlag = uint16(614);
            du: turningPWM = lineTracker(single(-0.3), normalizedLight, single(1.3), sensors.battery);
            state Vel3
            state Vel2
              du: des_vel = des_vel + single(0.00024);
            Vel2 -> Vel3 : [des_vel >= single(0.15)]
            (default) -> Vel2
          (default) -> JumpOnIt
          JumpOnIt -> GoingUP : [states.balancerStates.theta >= theta_ref+single(1.6)]
          MoveForward -> Wait : [sensors.BT_status_in == single(4)]
          Wait -> see_saw_mode.Balancing.SeesawLogic.Seesaw.Stop : [sensors.BT_status_in == single(5)] %[states.balancerStates.theta >= theta_ref + single(30)]
          see_saw_mode.Balancing.SeesawLogic.Seesaw.Stop -> RaceDone : [states.balancerStates.theta >= theta_ref + single(30)]
          RaceDone -> FoundLine [order 2] : [normalizedLight > single(0.4)]
        (default) -> StationnaryBalance
        StationnaryBalance -> Approach : [sensors.BT_status_in == single(2)]
        Detect -> Seesaw : [states.balancerStates.theta_dot<single(0)]
      state After [parallel]
        during:
        forwardPWM = balance_ctrl(states.balancerStates, des_vel ,sensors.battery)
        PWM.left = forwardPWM + turningPWM;
        PWM.right = forwardPWM - turningPWM;
        settings: executionOrder=2
    state cmd = lineTracker(desiredLight,light,trackingPower,battery) [function]
    state Speak [function]
    state cmd = tail_controller(current,desired) [function]
    state cmd = balance_ctrl(balancerStates,desired_velocity,battery) [function]
    state DispVar(Var) [function]
    state SitDown
      state Stop
        during:
        during:
        forwardPWM = balance_ctrl(states.balancerStates, des_vel ,sensors.battery)
        PWM.left = forwardPWM;
        PWM.right = forwardPWM;
        desired_tail = single(1.6); %radian
      state Kick
        entry:
        PWM.left = single(100)
        PWM.right = single(100);
        exit:
        PWM.left = single(0)
        PWM.right = single(0);
      state Done
        entry:
        debugFlag = uint16(402);
        PWM.left = single(0); PWM.right = single(0);
        %current_mode_status = OperationModeStatusEnum.SUCCESSFULLY_COMPLETED;
      (default) -> see_saw_mode.SitDown.Stop
      see_saw_mode.SitDown.Stop -> Kick : after(0.5,sec)
      Kick -> Done : after(0.2,sec)
    (default) -> Pause
    Pause -> StandUp : [sensors.BT_status_in == single(1)]
    StandUp -> Balancing : [desired_tail >=single(2.0) && sensors.theta_T >= single(2.0)]
    RaceDone -> SitDown [order 1] : [states.balancerStates.theta >= theta_ref + single(70)]
    FoundLine -> SitDown : [states.balancerStates.theta >= theta_ref + single(70)]
  data: rawLight function_input single size=1; lightCalib function_input Bus: Light_Bus size=1; light function_output; cmd function_output; phi function_input single size=1; desiredPhi function_input single size=1; battery function_input double size=1; cmd function_output single size=1; desiredLight function_input single size=1; light function_input single size=1; trackingPower function_input single size=1; battery function_input double size=1; current function_input single size=1; desired function_input single size=1; cmd function_output single size=1; balancerStates function_input Bus: Balancer_States_Bus size=1; desired_velocity function_input single size=1; battery function_input double size=1; cmd function_output single size=1; Var function_input single size=1; states input Bus: States_Bus size=1; sensors input Bus: Sensors_Bus size=1; PWM output Bus: PWM_bus size=1; initFlags output Bus: Init_Bus size=1; debugFlag output uint16 size=1; desired_states local Bus: Balancer_States_Bus size=1; desired_tail local single size=1; current_mode_status data_store_memory; balancerStates_Bus0 parameter Bus: Balancer_States_Bus size=1; lightCalib data_store_memory; normalizedLight local single size=1; des_vel local single size=1; theta_ref local single size=1; forwardPWM local single size=1; turningPWM local single size=1; BT_status_out output single size=1; phi0 local single size=1; desired_phi local single size=1; theta_ref_2 local
